simulink model "hho"  (R2022a)
settings: Solver=VariableStepAuto  StartTime=0.0  StopTime=1  RelTol=1e-3
libraries: spsSeriesRLCBranchLib x7, spsDiodeLib x4, spsStairGeneratorLib x4, spsVoltageMeasurementLib x3, spsPVArrayLib x3, spsCurrentMeasurementLib x2, spsGroundLib x1, spsMosfetLib x1, spsPWMGeneratorDCDCLib x1, spspowerguiLib x1
settings Model: Creator=msi  LastModifiedBy=msi

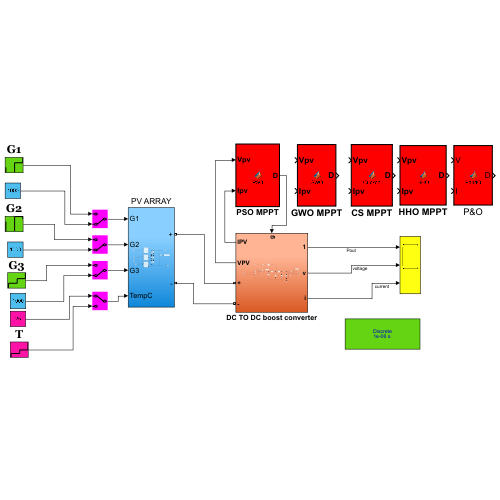
[thumbnail: Simulink's stored preview of the top-level diagram]
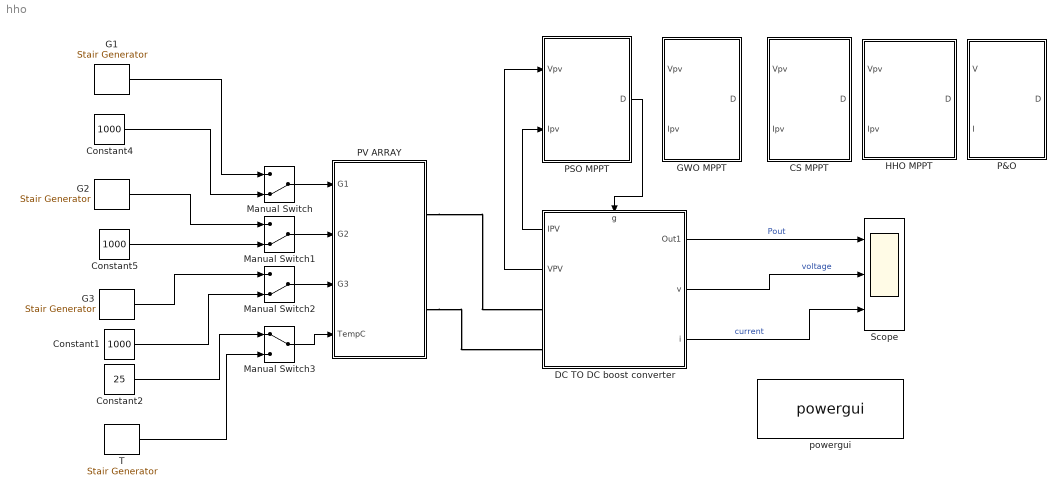
== system hho ==
  CS MPPT : MATLAB Function  TreatAsAtomicUnit=on
  Constant1 : Constant  Value=1000
  Constant2 : Constant  Value=25
  Constant4 : Constant  Value=1000
  Constant5 : Constant  Value=1000
  DC TO DC boost converter : Subsystem
      settings: PortSchema="{\"entries\":[{\"content\":{\"sides\":[{\"content\":{\"connectorIds\":[\"Out4\",\"Out5\",\"LConn1\",\"LConn2\"]},\"type\":\"ConnectorPlacement.EquallySpacedRectSide\",\"uuid\":\"bed9cabd-0612-41fc-bb5e-97f0075e7888\"},{\"content\":{\"connectorIds\":[\"Out1\",\"Out2\",\"Out3\"],\"side\":\"RIGHT\"},\"type\":\"ConnectorPlacement.EquallySpacedRectSide\",\"uuid\":\"934252dc-c08a-474d-9acc-ec5fd3ee8129\"},{\"content\":{\"connectorIds\":[\"In1\"],\"side\":\"TOP\"},\"type\":\"ConnectorPlacement.EquallySpacedRectSide\",\"uuid\":\"a6c96559-c135-4f10-8a5b-2290738f1393\"}]},\"type\":\"ConnectorPlacement.EquallySpacedConnector\",\"uuid\":\"b1692f17-bece-4195-a8f2-789748dd7599\"}],\"packageUris\":[\"http://schema.mathworks.com/mf0/Connector/R2020b\"],\"version\":\"1.0\"}"
  G1 : spsStairGeneratorLib/Stair Generator  t=[0, 0.5, 1.5, 2.5]  e=[800, 700, 900, 1000 ]  Ts=0
  G2 : spsStairGeneratorLib/Stair Generator  t=[0, 0.5, 1.5, 2.5]  e=[700, 500, 800, 750 ]  Ts=0
  G3 : spsStairGeneratorLib/Stair Generator  t=[0, 1, 2, 3]  e=[200, 400, 600, 850 ]  Ts=0
  GWO MPPT : MATLAB Function  TreatAsAtomicUnit=on
  HHO MPPT : MATLAB Function  TreatAsAtomicUnit=on
  Manual Switch : ManualSwitch  CurrentSetting=0
  Manual Switch1 : ManualSwitch  CurrentSetting=0
  Manual Switch2 : ManualSwitch  CurrentSetting=0
  Manual Switch3 : ManualSwitch
  P&O : MATLAB Function  TreatAsAtomicUnit=on
  PSO MPPT : MATLAB Function  TreatAsAtomicUnit=on
  PV ARRAY : Subsystem
  Scope : Scope  NumInputPorts=3
  T : spsStairGeneratorLib/Stair Generator  t=[0, 0.5, 1.5, 2.5]  e=[20 ,25, 30, 40 ]  Ts=0
  powergui : spspowerguiLib/powergui  Priority=1  SimulationMode=Discrete  SampleTime=1e-6  frequency=60  Iterations=50  frequencyindice=0  Pbase=100e6  ErrMax=1e-4  UnitsV=kV  UnitsW=MW  buscounter=0  FunctionMessages=off  echomessages=off  EnableUseOfTLC=off  CurrentSourceSwitches=off  DisableSnubberDevices=off  DisableRonSwitches=off  DisableVfSwitches=off  DisplayEquations=off  AutomaticDiscreteSolvers=off  SolverType=Backward Euler  Interpol=off  ExternalGateDelay=off  methode=off  Ts=0  x0status=blocks  SPID=on  SwTol=0  HookPort=off  NonlinearTolerance=1e-4  nMaxIteration=100  ContinueOnMaxIteration=off  RestoreLinks=warning  ResistiveCurrentMeasurement=off  Frange=[0:2:500]  Ylog=off  Xlog=on  ShowGrid=off  save=off  variable=ZData  structure=0  ZoomFFT=off  StartTime=0.0  cycles=1  DisplayStyle=1  fundamental=60  FreqAxis=off  MaxFrequency=1000  frequencyindicesteady=1  RmsSteady=1  display=off
  wires:
  Manual Switch/1 -> PV ARRAY/1(G1)
  DC TO DC boost converter/4(IPV) -> PSO MPPT/2(Ipv)
  DC TO DC boost converter/2(v) -> Scope/2  "voltage"
  DC TO DC boost converter/3(i) -> Scope/3  "current"
  DC TO DC boost converter/5(VPV) -> PSO MPPT/1(Vpv)
  Manual Switch1/1 -> PV ARRAY/2(G2)
  Manual Switch3/1 -> PV ARRAY/4(TempC)
  DC TO DC boost converter/1(Out1) -> Scope/1  "Pout"
  Manual Switch2/1 -> PV ARRAY/3(G3)
  PSO MPPT/1(D) -> DC TO DC boost converter/1(g)
  G3/1 -> Manual Switch2/1
  T/1 -> Manual Switch3/2
  Constant1/1 -> Manual Switch2/2
  G1/1 -> Manual Switch/1
  Constant5/1 -> Manual Switch1/2
  G2/1 -> Manual Switch1/1
  Constant2/1 -> Manual Switch3/1
  Constant4/1 -> Manual Switch/2
  connections:
  PV ARRAY/RConn1 -- DC TO DC boost converter/LConn1
  PV ARRAY/RConn2 -- DC TO DC boost converter/LConn2

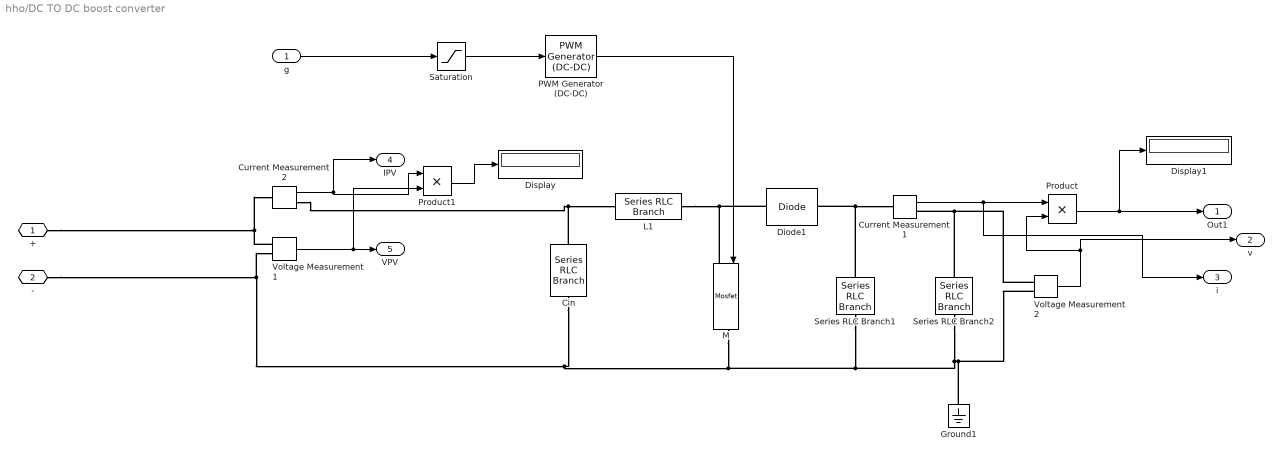
== system hho/DC TO DC boost converter ==
  g : Inport
  Cin : spsSeriesRLCBranchLib/Series RLC Branch  LConnTagsString=__new0  RConnTagsString=__new0  BranchType=C  Resistance=1e-3  Inductance=250e-6  SetiL0=off  InitialCurrent=0  Capacitance=72e-6  Setx0=off  InitialVoltage=0  Measurements=None
  Current Measurement1 : spsCurrentMeasurementLib/Current Measurement  PhasorSimulation=off  OutputType=Complex  PSBequivalent=0
  Current Measurement2 : spsCurrentMeasurementLib/Current Measurement  PhasorSimulation=off  OutputType=Complex  PSBequivalent=0
  Diode1 : spsDiodeLib/Diode  Ron=0.001  Lon=0  Vf=0.8  IC=0  UseSnubber=off  Rs=500  Cs=250e-9  Measurements=off
  Display : Display
  Display1 : Display
  Ground1 : spsGroundLib/Ground  LConnTagsString=a
  L1 : spsSeriesRLCBranchLib/Series RLC Branch  LConnTagsString=__new0  RConnTagsString=__new0  BranchType=L  Resistance=1e-3  Inductance=5.5e-3  SetiL0=off  InitialCurrent=0  Capacitance=1e-6  Setx0=off  InitialVoltage=0  Measurements=None
  M : spsMosfetLib/Mosfet  Ron=1e-3  Lon=0  Rd=1e-3  Vfd=0  IC=0  Rs=1e5  Cs=inf  Measurements=off
  PWM Generator (DC-DC) : spsPWMGeneratorDCDCLib/PWM Generator (DC-DC)  Fsw=5000  Ts=0
  Product : Product
  Product1 : Product
  Saturation : Saturate  UpperLimit=1  LowerLimit=0
  Series RLC Branch1 : spsSeriesRLCBranchLib/Series RLC Branch  LConnTagsString=__new0  RConnTagsString=__new0  BranchType=C  Resistance=1e-4  Inductance=200e-6  SetiL0=off  InitialCurrent=0  Capacitance=133e-6  Setx0=off  InitialVoltage=40  Measurements=None
  Series RLC Branch2 : spsSeriesRLCBranchLib/Series RLC Branch  LConnTagsString=__new0  RConnTagsString=__new0  BranchType=R  Resistance=60  Inductance=200e-6  SetiL0=off  InitialCurrent=0  Capacitance=75e-5  Setx0=off  InitialVoltage=40  Measurements=None
  Voltage Measurement1 : spsVoltageMeasurementLib/Voltage Measurement  PhasorSimulation=off  OutputType=Complex  PSBequivalent=0
  Voltage Measurement2 : spsVoltageMeasurementLib/Voltage Measurement  PhasorSimulation=off  OutputType=Complex  PSBequivalent=0
  + : PMIOPort  Side=Left
  - : PMIOPort  Port=2  Side=Left
  Out1 : Outport
  v : Outport  Port=2
  i : Outport  Port=3
  IPV : Outport  Port=4
  VPV : Outport  Port=5
  wires:
  Current Measurement1/1 -> i/1, Product/1
  Voltage Measurement2/1 -> v/1, Product/2
  Voltage Measurement1/1 -> Product1/2, VPV/1
  Product/1 -> Display1/1, Out1/1
  g/1 -> Saturation/1
  PWM Generator (DC-DC)/1 -> M/1
  Saturation/1 -> PWM Generator (DC-DC)/1
  Current Measurement2/1 -> IPV/1, Product1/1
  Product1/1 -> Display/1
  connections:
  M/RConn1 -- Series RLC Branch1/LConn1 -- Ground1/LConn1 -- Voltage Measurement2/LConn2 -- Series RLC Branch2/RConn1 -- Cin/LConn1 -- -/RConn1 -- Voltage Measurement1/LConn2
  Voltage Measurement1/LConn1 -- +/RConn1 -- Current Measurement2/LConn1
  Series RLC Branch1/RConn1 -- Diode1/RConn1 -- Current Measurement1/LConn1
  Voltage Measurement2/LConn1 -- Series RLC Branch2/LConn1 -- Current Measurement1/RConn1
  Current Measurement2/RConn1 -- Cin/RConn1 -- L1/LConn1
  L1/RConn1 -- Diode1/LConn1 -- M/LConn1

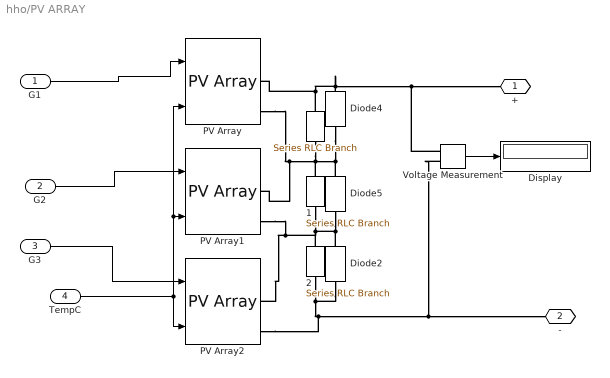
== system hho/PV ARRAY ==
  G1 : Inport
  G2 : Inport  Port=2
  G3 : Inport  Port=3
  TempC : Inport  Port=4
  " " : spsSeriesRLCBranchLib/Series RLC Branch  LConnTagsString=__new0  RConnTagsString=__new0  BranchType=C  Resistance=1e-3  Inductance=250e-6  SetiL0=off  InitialCurrent=0  Capacitance=10e-6  Setx0=off  InitialVoltage=0  Measurements=None
  " 1" : spsSeriesRLCBranchLib/Series RLC Branch  LConnTagsString=__new0  RConnTagsString=__new0  BranchType=C  Resistance=1e-3  Inductance=250e-6  SetiL0=off  InitialCurrent=0  Capacitance=10e-6  Setx0=off  InitialVoltage=0  Measurements=None
  " 2" : spsSeriesRLCBranchLib/Series RLC Branch  LConnTagsString=__new0  RConnTagsString=__new0  BranchType=C  Resistance=1e-3  Inductance=250e-6  SetiL0=off  InitialCurrent=0  Capacitance=10e-6  Setx0=off  InitialVoltage=0  Measurements=None
  Diode2 : spsDiodeLib/Diode  Ron=0.001  Lon=0  Vf=0.5  IC=0  UseSnubber=off  Rs=500  Cs=250e-9  Measurements=off
  Diode4 : spsDiodeLib/Diode  Ron=0.001  Lon=0  Vf=0.5  IC=0  UseSnubber=off  Rs=500  Cs=250e-9  Measurements=off
  Diode5 : spsDiodeLib/Diode  Ron=0.001  Lon=0  Vf=0.5  IC=0  UseSnubber=off  Rs=500  Cs=250e-9  Measurements=off
  Display : Display
  PV Array : spsPVArrayLib/PV Array  Npar=1  Nser=1  PlotType=array @ 1000 W/m2 & specified temperatures  S_vec="[ 1000  500  100 ]"  Temp_C_vec="[ 45 25  ]"  ModuleName=Kyocera Solar KD320GX-LPB  PlotWhenSelected=off  Pm=320.399  Ncell=80  Voc=49.5  Isc=8.6  Vm=40.1  Im=7.99  beta_Voc_pc=-0.3624  alpha_Isc_pc=0.071  beta_Voc=-0.17939  alpha_Isc=0.006106  IL=8.6153  I0=3.2022e-10  nI=1.0039  Rsh=233.3987  Rs=0.41435  RobustModel=off  RobustCellTemperature=313.3991  BAL=on  Tc=1e-6  Tfilter=5e-5
  PV Array1 : spsPVArrayLib/PV Array  Npar=1  Nser=1  PlotType=array @ 1000 W/m2 & specified temperatures  S_vec="[ 1000  500  100 ]"  Temp_C_vec="[ 45 25  ]"  ModuleName=Kyocera Solar KD320GX-LPB  PlotWhenSelected=off  Pm=320.399  Ncell=80  Voc=49.5  Isc=8.6  Vm=40.1  Im=7.99  beta_Voc_pc=-0.3624  alpha_Isc_pc=0.071  beta_Voc=-0.17939  alpha_Isc=0.006106  IL=8.6153  I0=3.2022e-10  nI=1.0039  Rsh=233.3987  Rs=0.41435  RobustModel=off  RobustCellTemperature=313.3991  BAL=on  Tc=1e-6  Tfilter=5e-5
  PV Array2 : spsPVArrayLib/PV Array  Npar=1  Nser=1  PlotType=array @ 1000 W/m2 & specified temperatures  S_vec="[ 1000  500  100 ]"  Temp_C_vec="[ 45 25  ]"  ModuleName=Kyocera Solar KD320GX-LPB  PlotWhenSelected=off  Pm=320.399  Ncell=80  Voc=49.5  Isc=8.6  Vm=40.1  Im=7.99  beta_Voc_pc=-0.3624  alpha_Isc_pc=0.071  beta_Voc=-0.17939  alpha_Isc=0.006106  IL=8.6153  I0=3.2022e-10  nI=1.0039  Rsh=233.3987  Rs=0.41435  RobustModel=off  RobustCellTemperature=313.3991  BAL=on  Tc=1e-6  Tfilter=5e-5
  Voltage Measurement : spsVoltageMeasurementLib/Voltage Measurement  PhasorSimulation=off  OutputType=Complex  PSBequivalent=0
  + : PMIOPort  Side=Right
  - : PMIOPort  Port=2  Side=Right
  wires:
  TempC/1 -> PV Array2/2, PV Array1/2, PV Array/2
  G1/1 -> PV Array/1
  G3/1 -> PV Array2/1
  G2/1 -> PV Array1/1
  Voltage Measurement/1 -> Display/1
  connections:
  Diode4/RConn1 -- PV Array/RConn1 -- " "/LConn1 -- Voltage Measurement/LConn1 -- +/RConn1
  Diode2/LConn1 -- " 2"/RConn1 -- PV Array2/RConn2 -- Voltage Measurement/LConn2 -- -/RConn1
  Diode5/RConn1 -- PV Array1/RConn1 -- PV Array/RConn2 -- " 1"/LConn1 -- " "/RConn1 -- Diode4/LConn1
  Diode5/LConn1 -- " 2"/LConn1 -- " 1"/RConn1 -- PV Array2/RConn1 -- PV Array1/RConn2 -- Diode2/RConn1

== matlab function hho/HHO MPPT ==
  settings: updateMethod=DISCRETE  sampleTime=1e-4
  data: Vpv input; D output; Ipv input
function D = HHO( Vpv,Ipv)
%#codegen
persistent u;
persistent dcurrent;
persistent pbest;
persistent p;
persistent dc;
persistent v;
persistent counter;
persistent gbest;
persistent bbest;
persistent CC;
persistent mean_d;
persistent nHourse;
P=Vpv*Ipv;
if(isempty(counter))
    counter=0;
end
if(isempty(dcurrent))
    dcurrent=0.5;
end
if(isempty(gbest))
    gbest=0.5;
    bbest=0.1;
    CC=1;
    mean_d=0;
end
if(isempty(p))
    p=zeros(4,1);
end

if(isempty(v))
    v=zeros(4,1);
end

if(isempty(pbest))
    pbest=zeros(4,1);
end
if(isempty(u))
    u=0;
end
if(isempty(dc))
    dc=zeros(4,1);
    dc(1)=0;
    dc(2)=0.2;
    dc(3)=0.4;
    dc(4)=0.7;
    nHourse=length(dc);
end

if(counter>=1 && counter<300)
    D=dcurrent;
    counter=counter+1;
    return;
end
counter=0;
  
if(u>=1 && u<=4)
    if((Vpv*Ipv)>p(u))
        p(u)=Vpv*Ipv;
        pbest(u)=dcurrent;
    end
end
u=u+1;
if(u==6)
    u=1;
end
if(u==1)
    D=dc(u);
    dcurrent=D;
    counter=1;
    return;
elseif(u==2)
    D=dc(u);
    dcurrent=D;
    counter=1;
    return;
elseif(u==3)
    D=dc(u);
    dcurrent=D;
    counter=1;
    return;
elseif(u==4)
    D=dc(u);
    dcurrent=D;
    counter=1;
    return;
elseif(u==5 )

    [m,i]=max(p);
    [mi,jj]=min(p);
    gbest=pbest(i);
    bbest=pbest(jj);
    D=gbest;
    dcurrent=D;
    counter=1;
    pp=[1;2;3;4];
    xxx=[pp p];
    ii=sortrows(xxx,2);
    CC=find(ii==1);
    mean_d=mean(dc);
    nHourse=length(dc);
    %update velocity and duty cycle
    v(1)=updatevelocity(v(1),pbest(1),dc(1),gbest,bbest,CC,mean_d,nHourse);
    CC=find(ii==2);
    v(2)=updatevelocity(v(2),pbest(2),dc(2),gbest,bbest,CC,mean_d,nHourse);
    CC=find(ii==3);
    v(3)=updatevelocity(v(3),pbest(3),dc(3),gbest,bbest,CC,mean_d,nHourse);
    CC=find(ii==4);
    v(4)=updatevelocity(v(4),pbest(4),dc(4),gbest,bbest,CC,mean_d,nHourse);
    %update duty cycle
    dc(1)=updateduty(dc(1),v(1));
    dc(2)=updateduty(dc(2),v(2));
    dc(3)=updateduty(dc(3),v(3));
    dc(4)=updateduty(dc(4),v(4));
    
    return;
    
else
    u
    y='hello'
    D=0.1
    
end


end
function vfinal=updatevelocity(velocity,pobest,d,gwbest,bbbest,cc,md,nh)
vfinal=velocity;
goodp=(gwbest+bbbest)/2;
w=1;
phiD=0.02;
phiI=0.02;
xx=0.8;

g_Alpha=xx*1.50;       % Grazing
d_Alpha=xx*0.5;        % Defense Mechanism
h_Alpha=xx*1.5;        % Hierarchy

g_Beta=xx*1.50;       % Grazing
h_Beta=xx*0.9;        % Hierarchy 
s_Beta=xx*0.20;       % Sociability
d_Beta=xx*0.20;       % Defense Mechanism

g_Gamma=xx*1.50;       % Grazing 
h_Gamma=xx*0.50;       % Hierarchy 
s_Gamma=xx*0.10;        % Sociability 
i_Gamma=xx*0.30;       % Imitation
d_Gamma=xx*0.10;       % Defense Mechanism 
r_Gamma=xx*0.05;       % Random (Wandering and Curiosity)

g_Delta=xx*1.50;       % Grazing
r_Delta=xx*0.10;       % Random (Wandering and Curiosity)

c1=0.2;
c2=1.3;
w=0.1;
cc;
if cc<=0.1*nh
vfinal = +h_Alpha*rand*(gwbest-d)-d_Alpha*rand*d+g_Alpha*(0.95+0.1*rand)*(pobest-d);
elseif cc<=0.3*nh
vfinal = +s_Beta*rand*(md-d)-d_Beta*rand*(bbbest-d)+h_Beta*rand*(gwbest-d)+g_Beta*(0.95+0.1*rand)*(pobest-d);
elseif cc<=0.6*nh
vfinal = +s_Gamma*rand*(md-d)+r_Gamma*rand*d-d_Gamma*rand*(bbbest-d)+h_Gamma*rand*(gwbest-d)+i_Gamma*rand*(goodp-d)+g_Gamma*(0.95+0.1*rand)*(pobest-d);
else
vfinal = +r_Delta*rand*d+g_Delta*(0.95+0.1*rand)*(pobest-d);   
end
end
function dfinal=updateduty(d,velocity)
w=1.2;
dup=d+w*velocity;
if(dup>1)
    dfinal=1;
elseif(dup<0.1)
    dfinal=0.1;
else
    dfinal=dup;
end
end

== matlab function hho/CS MPPT ==
  settings: updateMethod=DISCRETE  sampleTime=1e-4
  data: Vpv input; D output; Ipv input
function D = Cuckoo(Vpv,Ipv)
%#codegen
persistent u;
persistent dcurrent;
persistent p;
persistent dc;
persistent dbest;
persistent counter;
persistent iworst;
persistent discover;
if(isempty(discover))
    discover=0;
end
if(isempty(counter))
    counter=0;
end
if(isempty(dcurrent))
    dcurrent=0.5;
end
if(isempty(iworst))
    iworst=0;
end



if(isempty(dbest))
    dbest=0;
end
if(isempty(p))
    p=zeros(4,1);
end
if(isempty(u))
    u=0;
end
if(isempty(dc))
    dc=zeros(4,1);
    dc(1)=0;
    dc(2)=0.3;
    dc(3)=0.5;
    dc(4)=0.9;
end
if(counter>=1 && counter<150)
    D=dcurrent;
    counter=counter+1;
    return;
end
counter=0;

if(u>=1 && u<=4)
    p(u)=Vpv*Ipv;
end
u=u+1;
if(u==7)
    u=1;
end
if(u==1)
    D=dc(u);
    dcurrent=D;
    counter=1;
    return;
elseif(u==2)
    D=dc(u);
    dcurrent=D;
    counter=1;
    return;
elseif(u==3)
    D=dc(u);
    dcurrent=D;
    counter=1;
    return;
elseif(u==4)
    D=dc(u);
    dcurrent=D;
    counter=1;
    return;
elseif(u==5 || u==6 )
    if(u==5)
        if(rand(1)>0.25)
            discover=1;
            [m,i]=max(p)
            dbest=dc(i);
            %determine the worst nest
            [m,iworst]=min(p);
            %build new nest
            %dc(iworst)=dbest;
            dc(iworst)=levyflight(dbest,dc(iworst));
            %dc(iworst)=withinlimits(dc(iworst));
            D=dc(iworst);
            dcurrent=D;
            counter=1;
            return;
        else
            u=u+1;
            [m,i]=max(p)
            dbest=dc(i);
            D=dbest;
            dcurrent=D;
            counter=1;
            dc(1)=levyflight(dbest,dc(1))
            % dc(1)=withinlimits(dc(1))
            dc(2)=levyflight(dbest,dc(2))
            %dc(2)=withinlimits(dc(2))
            dc(3)=levyflight(dbest,dc(3))
            % dc(3)=withinlimits(dc(3))
            dc(4)=levyflight(dbest,dc(4))
            % dc(4)=withinlimits(dc(4))
            return;
        end
        
    else
        %calculate new power of new nest
        p(iworst)=Vpv*Ipv;
        %determine the best nest
        [m,i]=max(p);
        dbest=dc(i);
        D=dbest;
        dcurrent=D;
        counter=1;
        
        dc(1)=levyflight(dbest,dc(1))
        % dc(1)=withinlimits(dc(1))
        dc(2)=levyflight(dbest,dc(2))
        %dc(2)=withinlimits(dc(2))
        dc(3)=levyflight(dbest,dc(3))
        % dc(3)=withinlimits(dc(3))
        dc(4)=levyflight(dbest,dc(4))
        % dc(4)=withinlimits(dc(4))
        discover=0;
        return;
    end
    
else
    u
    y='hello'
    D=0.1
    
end


end
function dfinal=levyflight(dbest,d)
beta=3/2;
kcoeff=0.9;
sigmau=(gamma(1+beta)*sin(pi*beta/2)/(gamma((1+beta)/2)*beta*2^((beta-1)/2)))^(1/beta);
sigmav=1;
u=normrnd(0,(sigmau)^2);
v=normrnd(0,(sigmav)^2);
dup=d+(kcoeff*(abs(u)/((abs(v))^(1/beta)))*(dbest-d));


if(dup>1)
    dfinal=1;
elseif(dup<0)
    dfinal=0;
else
    dfinal=dup;
end
end

== matlab function hho/PSO MPPT ==
  settings: updateMethod=DISCRETE  sampleTime=1e-4
  data: Vpv input; D output; Ipv input
function D = PSO(Vpv,Ipv)
%#codegen
persistent u;
persistent dcurrent;
persistent pbest;
persistent p;
persistent dc;
persistent v;
persistent counter;
persistent gbest;
if(isempty(counter))
    counter=0;
end
if(isempty(dcurrent))
    dcurrent=0.9;
end
if(isempty(gbest))
    gbest=0.9;
end
if(isempty(p))
    p=zeros(4,1);
end

if(isempty(v))
    v=zeros(4,1);
end

if(isempty(pbest))
    pbest=zeros(4,1);
end
if(isempty(u))
    u=0;
end
if(isempty(dc))
    dc=zeros(4,1);
    dc(1)=0;
    dc(2)=0.1;
    dc(3)=0.4;
    dc(4)=0.7;
end
if(counter>=1 && counter<300)
    D=dcurrent;
    counter=counter+1;
    return;
end
counter=0;

if(u>=1 && u<=4)
    if((Vpv*Ipv)>p(u))
        p(u)=Vpv*Ipv;
        pbest(u)=dcurrent;
    end
end
u=u+1;
if(u==6)
    u=1;
end
if(u==1)
    D=dc(u);
    dcurrent=D;
    counter=1;
    return;
elseif(u==2)
    D=dc(u);
    dcurrent=D;
    counter=1;
    return;
elseif(u==3)
    D=dc(u);
    dcurrent=D;
    counter=1;
    return;
elseif(u==4)
    D=dc(u);
    dcurrent=D;
    counter=1;
    return;
elseif(u==5 )
    [m,i]=max(p);
    gbest=pbest(i);
    D=gbest;
    dcurrent=D;
    counter=1;
    %update velocity and duty cycle
    v(1)=updatevelocity(v(1),pbest(1),dc(1),gbest);
    v(2)=updatevelocity(v(2),pbest(2),dc(2),gbest);
    v(3)=updatevelocity(v(3),pbest(3),dc(3),gbest);
    v(4)=updatevelocity(v(4),pbest(4),dc(4),gbest);
    %update duty cycle
    dc(1)=updateduty(dc(1),v(1));
    dc(2)=updateduty(dc(2),v(2));
    dc(3)=updateduty(dc(3),v(3));
    dc(4)=updateduty(dc(4),v(4));
    
    return;
    
else
    u
    y='hello'
    D=0.1
    
end


end
function vfinal=updatevelocity(velocity,pobest,d,gwbest)
% PSO Parameters
w=0.1;
%w=(1.1-(pobest/gwbest));            % Inertia Weight
             % Inertia Weight Damping Ratio
c1=0.2;         % Personal Learning Coefficient
c2=1.3;         % Global Learning Coefficient

% If you would like to use Constriction Coefficients for PSO,
% uncomment the following block and comment the above set of parameters.

% % Constriction Coefficients
% phi1=2.05;
% phi2=2.05;
% phi=phi1+phi2;
% chi=2/(phi-2+sqrt(phi^2-4*phi));
% w=chi;          % Inertia Weight
% wdamp=1;        % Inertia Weight Damping Ratio
% c1=chi*phi1;    % Personal Learning Coefficient
% c2=chi*phi2;    % Global Learning Coefficient
vfinal = (w*velocity)+(c1*rand(1)*(pobest-d))+(c2*rand(1)*(gwbest-d));
end
function dfinal=updateduty(d,velocity)
dup=d+velocity;
if(dup>1)
    dfinal=1;
elseif(dup<0.1)
    dfinal=0.1;
else
    dfinal=dup;
end
end

== matlab function hho/P&O ==
  settings: updateMethod=DISCRETE
  data: D output; V input; I input
% author : Saad MOTAHHIR
% f =50000 hz (G)
function D  = PandO(V, I)


Dinit = 0.1;  %Initial value for D output
Dmax = 0.8;   %Maximum value for D
Dmin = 0.1;   %Minimum value for D
deltaD = 0.0001; %Increment value used to increase/decrease the duty cycle D


persistent Vold Pold Dold;

dataType = 'double';

if isempty(Vold)
    Vold=0;
    Pold=0;
    Dold=Dinit;
end
P= V*I;
dV= V - Vold;
dP= P - Pold;

    if dP < 0
        if dV < 0
            D = Dold - deltaD;
        else
            D = Dold + deltaD;
        end
    else
        if dV < 0
            D = Dold + deltaD;
        else
            D = Dold - deltaD;
        end    
    end

if D >= Dmax | D<= Dmin
    D=Dold;
end

Dold=D;
Vold=V;
Pold=P;

== matlab function hho/GWO MPPT ==
  settings: updateMethod=DISCRETE  sampleTime=1e-4
  data: Vpv input; D output; Ipv input
function D = GWO(Vpv,Ipv)
%#codegen
persistent u;
persistent dcurrent;
persistent p pc;
persistent dc dcheck;
persistent dbest dworst;
persistent counter iteration;
persistent iworst;
persistent deltad;
persistent Fk;
persistent En alpha beta_pos delta_pos alpha_pos beta_score delta_score;
if(isempty(alpha))
    alpha=0;
end
if(isempty(beta_pos))
    alpha_pos= zeros(1, 1);
    beta_pos= zeros(1, 1);
    delta_pos= zeros(1, 1);
    beta_score=0;
    delta_score =0;
end
if(isempty(iteration))
iteration=0;
end
if(isempty(counter))
    counter=0;
end
if(isempty(dcurrent))
    dcurrent=0.5;
end
if(isempty(iworst))
    iworst=0;
    dworst=0;
end
if(isempty(deltad))
    deltad=zeros(4,1);
end
if(isempty(Fk))
    Fk=zeros(4,1);
end
if(isempty(En))
    En=zeros(4,1);
end
if(isempty(dbest))
    dbest=0;
    best=0;
end
if(isempty(p))
    p=zeros(4,1);
    pc=zeros(3,1);
   
end
if(isempty(u))
    u=0;
end
if(isempty(dc))
    dc=zeros(4,1);
    dcheck=zeros(3,1);
    dc(1)=0.16;
    dc(2)=0.34;
    dc(3)=0.51;
    dc(4)=0.71;
end
  
if(counter>=1 && counter<200)
   
    if(u>=1 && u<=4)
       p(u)=Vpv*Ipv;
    end
 D=dcurrent;
    counter=counter+1;
    return;
end
counter=0;
 
 
u=u+1;
if(u==6)
    u=1;
end
 
if(u==1)
    D=dc(u);
    dcurrent=D;
    counter=1;
  
  
    return;
elseif(u==2)
    D=dc(u);
    dcurrent=D;
    counter=1;
 
    
    return;
elseif(u==3)
    D=dc(u);
    dcurrent=D;
    counter=1;
 
     
    return;
elseif(u==4)
    D=dc(u);
    dcurrent=D;
    counter=1;
 
    
    return;
elseif(u==5)
    iteration=iteration+1;
            for i=1:4
               Flag4ub=dc(i,:)>1;
               Flag4lb=dc(i,:)<0;
               dc(i)=(dc(i).*(~(Flag4ub+Flag4lb)))+1.*Flag4ub;
            end
            for ii=1:3
            [m,i]=max(p);
            dcheck(ii)=dc(i);
            pc(ii)=m;
            p(i)=0;
            end
            if(pc(1)>alpha)
                alpha=pc(1);
                alpha_pos=dcheck(1);
            end
         if(pc(2)>beta_score)
                beta_score=pc(2);
                beta_pos=dcheck(2);
         end
            if(pc(3)>delta_score)
                delta_score=pc(3);
                delta_pos=dcheck(3);
            end
            if(iteration<=5)
    dc1=pos_up(iteration,alpha_pos,dc,beta_pos,delta_pos);
    dc=dc1;    
            else
                dc(1)=alpha_pos;
                dc(2)=alpha_pos;
                dc(3)=alpha_pos;
                dc(4)=alpha_pos;
            end
            D=alpha_pos;
            dcurrent=D;
            counter=1;
       
      
          
            return;
else
    u;
    y='hello';
    D=0.1;
    
end
 
 
end
function D1=pos_up(l,alpha_pos,D_cur,beta_pos,delta_pos)
if(l>=5)
    l=5;
end
a=2-2*(l/5);
D1=zeros(4,1);
 
for kk=1:4
   r1=rand();
   r2=rand();
    A1=2*a*r1-a;
    C1=2*r2;
    D_alpha=abs(C1*alpha_pos-D_cur(kk));
    X1=alpha_pos-A1*D_alpha;
     r1=rand();
   r2=rand();
    A2=2*a*r1-a;
    C2=2*r2;
    D_beta=abs(C2*beta_pos-D_cur(kk));
    X2=beta_pos-A2*D_beta;
    r1=rand();
   r2=rand();
    A3=2*a*r1-a;
    C3=2*r2;
    D_delta=abs(C3*delta_pos-D_cur(kk));
    X3=delta_pos-A3*D_delta;
    
    X4=(X1+X2+X3)/3;
    D1(kk)=X4;
    if(D1(kk)>0.95)
        D1(kk)=0.55;
    elseif (D1(kk)<0.01)
        D1(kk)=0.51;
    end
end
disp(D1);
end
